simulink model "Prj2CDig"  (R2026a)
settings: Solver=ode45  StopTime=3600  RelTol=1e-6  EnableMultiTasking=on
values from neighbouring files (symbols this model uses):
  A = (Tz-Tp1)/(Tp2-Tp1)    (= 0.157044591698)    [Prj2CDig_m.m]
  B = 1 - A    (= 0.842955408302)    [Prj2CDig_m.m]
  K = Ka(1:2)    [Prj2CDig_m.m]
  Ki = -Ka(3)    [Prj2CDig_m.m]
  Kp = 0.8864/256.0    (= 0.0034625)    [Prj2CDig_m.m]
  L = acker(Aa',Ca',o)    [Prj2CDig_m.m]
  Nb = -Ki/p(1)    [Prj2CDig_m.m]
  PO = 60    [Prj2CDig_m.m]
  Ta = 27.4    [Prj2CDig_m.m]
  Tp1 = 323.16    [Prj2CDig_m.m]
  Tp2 = 37.636    [Prj2CDig_m.m]
  w0 = 0.09817477042468    (= 0.0981747704247)    [Prj2CDig_m.m]
  x1ei = 0    [Prj2CDig_m.m]
  x1i = 0    [Prj2CDig_m.m]
  x2ei = 0    [Prj2CDig_m.m]
  x2i = 0    [Prj2CDig_m.m]
  xii = 0    [Prj2CDig_m.m]
  xs1i = 0    [Prj2CDig_m.m]
  xs2i = 0    [Prj2CDig_m.m]
settings Model: Creator=Adolfo  LastModifiedBy=pedro
settings SolverCC: ZeroCrossControl=DisableAll
settings DataIOCC: MaxDataPoints=25000  SignalLoggingSaveFormat=ModelDataLogs
settings OptimizationCC: BooleanDataType=off  InitFltsAndDblsToZero=on
settings DebuggingCC: SaveWithParameterizedLinksMsg=none  UnderspecifiedInitializationDetection=Classic  SignalResolutionControl=TryResolveAllWithWarning  MultiTaskDSMMsg=warning  MultiTaskCondExecSysMsg=none
settings HardwareCC: ProdHWDeviceType=32-bit Generic  TargetUnknown=on
settings GRTTargetCC: TargetFcnLib=ansi_tfl_tmw.mat  CombineOutputUpdateFcns=off  GRTInterface=on

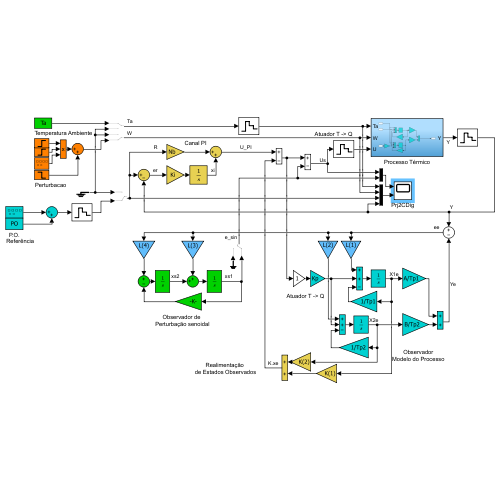
[thumbnail: Simulink's stored preview of the top-level diagram]
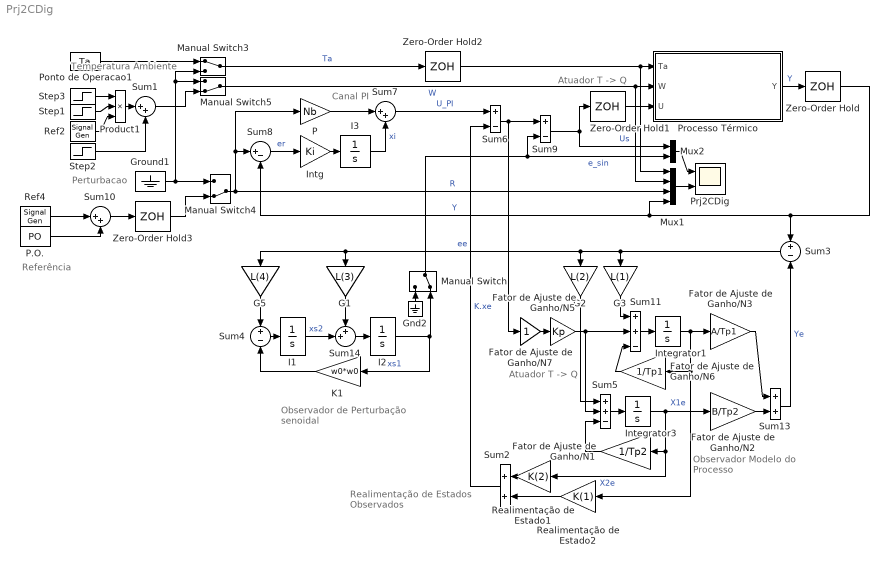
== system Prj2CDig ==
  note: Temperatura Ambiente
  note: Atuador T -> Q
  note: Referência
  note: Perturbacao
  note: Realimentação
      | de Estados Observados
  note: Observador de
      | Perturbação senoidal
  note: Observador
      | Modelo do Processo
  note: Canal PI
  note: Atuador T -> Q
  Fator de Ajuste de Ganho/N1 : Gain  Gain=1/Tp2  SaturateOnIntegerOverflow=on  OutDataTypeStr=Inherit: Same as input  ParamDataTypeStr=Inherit: Same as input
  Fator de Ajuste de Ganho/N2 : Gain  Gain=B/Tp2  SaturateOnIntegerOverflow=on  OutDataTypeStr=Inherit: Same as input  ParamDataTypeStr=Inherit: Same as input
  Fator de Ajuste de Ganho/N3 : Gain  Gain=A/Tp1  SaturateOnIntegerOverflow=on  OutDataTypeStr=Inherit: Same as input  ParamDataTypeStr=Inherit: Same as input
  Fator de Ajuste de Ganho/N5 : Gain  Gain=Kp  SaturateOnIntegerOverflow=on  OutDataTypeStr=Inherit: Same as input  ParamDataTypeStr=Inherit: Same as input
  Fator de Ajuste de Ganho/N6 : Gain  Gain=1/Tp1  SaturateOnIntegerOverflow=on  OutDataTypeStr=Inherit: Same as input  ParamDataTypeStr=Inherit: Same as input
  Fator de Ajuste de Ganho/N7 : Gain  SaturateOnIntegerOverflow=on  OutDataTypeStr=Inherit: Same as input  ParamDataTypeStr=Inherit: Same as input
  G1 : Gain  Gain=L(3)  SaturateOnIntegerOverflow=on  OutDataTypeStr=Inherit: Same as input  ParamDataTypeStr=Inherit: Same as input
  G2 : Gain  Gain=L(2)  SaturateOnIntegerOverflow=on  OutDataTypeStr=Inherit: Same as input  ParamDataTypeStr=Inherit: Same as input
  G3 : Gain  Gain=L(1)  SaturateOnIntegerOverflow=on  OutDataTypeStr=Inherit: Same as input  ParamDataTypeStr=Inherit: Same as input
  G5 : Gain  Gain=L(4)  SaturateOnIntegerOverflow=on  OutDataTypeStr=Inherit: Same as input  ParamDataTypeStr=Inherit: Same as input
  Gnd2 : Ground
  Ground1 : Ground
  I1 : Integrator  InitialCondition=xs2i
  I2 : Integrator  InitialCondition=xs1i
  I3 : Integrator  InitialCondition=xii
  Integrator1 : Integrator  InitialCondition=x1ei
  Integrator3 : Integrator  InitialCondition=x2ei
  Intg : Gain  Gain=Ki
  K1 : Gain  Gain=w0*w0  SaturateOnIntegerOverflow=on  OutDataTypeStr=Inherit: Same as input  ParamDataTypeStr=Inherit: Same as input
  Manual Switch : ManualSwitch  CurrentSetting=0
  Manual Switch3 : ManualSwitch
  Manual Switch4 : ManualSwitch  CurrentSetting=0
  Manual Switch5 : ManualSwitch  CurrentSetting=0
  Mux1 : Mux
  Mux2 : Mux  Inputs=2
  P : Gain  Gain=Nb
  P.O. : Constant  Value=PO
  Ponto de Operacao1 : Constant  Value=Ta
  Prj2CDig : Scope  NumInputPorts=2
      settings: TimeSpan=3600  ActiveDisplayYMinimum=-36403.221663907687  ActiveDisplayYMaximum=68827.440486001709  DataLoggingMaxPoints=30000
  Processo Térmico : Subsystem
  Product1 : Product  Inputs=3  RndMeth=Zero
  Realimentação de Estado1 : Gain  Gain=K(2)  SaturateOnIntegerOverflow=on  OutDataTypeStr=Inherit: Same as input  ParamDataTypeStr=Inherit: Same as input
  Realimentação de Estado2 : Gain  Gain=K(1)  SaturateOnIntegerOverflow=on  OutDataTypeStr=Inherit: Same as input  ParamDataTypeStr=Inherit: Same as input
  Ref2 : SignalGenerator  Frequency=w0  Units=rad/sec
  Ref4 : SignalGenerator  WaveForm=square  Amplitude=5  Frequency=.00125
  Step1 : Step  Time=3000  InitialValue=-20  FinalValue=0  SampleTime=0
  Step2 : Step  Time=1000  FinalValue=-20  SampleTime=0
  Step3 : Step  Time=1800  SampleTime=0
  Sum1 : Sum  Inputs=|++
  Sum10 : Sum  Inputs=|++
  Sum11 : Sum  Inputs=++-
  Sum13 : Sum  InputSameDT=on  SaturateOnIntegerOverflow=on  OutDataTypeStr=Inherit: Same as first input
  Sum14 : Sum  Inputs=++|  InputSameDT=on  SaturateOnIntegerOverflow=on  OutDataTypeStr=Inherit: Same as first input
  Sum2 : Sum
  Sum{3..4,6,9} (4 alike) : Sum  Inputs=+-  InputSameDT=on  SaturateOnIntegerOverflow=on  OutDataTypeStr=Inherit: Same as first input
  Sum5 : Sum  Inputs=++-
  Sum7 : Sum  Inputs=|++
  Sum8 : Sum  Inputs=|+-
  Zero-Order Hold{,1..3} (4 alike) : ZeroOrderHold  SampleTime=5
  wires:
  Sum9/1 -> Zero-Order Hold1/1, Mux2/1  "Us"
  P.O./1 -> Sum10/2
  Intg/1 -> I3/1
  Sum8/1 -> Intg/1  "er"
  P/1 -> Sum7/1
  I3/1 -> Sum7/2  "xi"
  Zero-Order Hold1/1 -> Processo Térmico/3(U)
  Manual Switch5/1 -> Mux1/2, Processo Térmico/2(W)  "W"
  Manual Switch3/1 -> Zero-Order Hold2/1  "Ta"
  Ground1/1 -> Manual Switch3/2, Manual Switch5/1, Manual Switch4/1
  Manual Switch4/1 -> Sum8/1, P/1, Mux1/3  "R"
  Sum1/1 -> Manual Switch5/2
  Ponto de Operacao1/1 -> Manual Switch3/1
  Sum10/1 -> Zero-Order Hold3/1
  Step2/1 -> Sum1/2
  Product1/1 -> Sum1/1
  Zero-Order Hold/1 -> Sum3/1, Sum8/2, Mux1/4  "Y"
  Fator de Ajuste de Ganho/N1/1 -> Sum5/3
  Integrator1/1 -> Fator de Ajuste de Ganho/N3/1, Fator de Ajuste de Ganho/N6/1, Realimentação de Estado2/1  "X1e"
  Manual Switch/1 -> Mux2/2, Sum9/2  "e_sin"
  Sum2/1 -> Sum6/2  "K.xe"
  Fator de Ajuste de Ganho/N6/1 -> Sum11/3
  Sum3/1 -> G5/1, G1/1, G2/1, G3/1  "ee"
  K1/1 -> Sum4/2
  Realimentação de Estado1/1 -> Sum2/1
  G5/1 -> Sum4/1
  I2/1 -> Manual Switch/2, K1/1  "xs1"
  Sum11/1 -> Integrator1/1
  Fator de Ajuste de Ganho/N2/1 -> Sum13/2
  Realimentação de Estado2/1 -> Sum2/2
  Sum5/1 -> Integrator3/1
  G3/1 -> Sum11/1
  Integrator3/1 -> Fator de Ajuste de Ganho/N2/1, Fator de Ajuste de Ganho/N1/1, Realimentação de Estado1/1  "X2e"
  Sum4/1 -> I1/1
  G2/1 -> Sum5/1
  Sum7/1 -> Sum6/1  "U_PI"
  Fator de Ajuste de Ganho/N5/1 -> Sum5/2, Sum11/2
  Sum14/1 -> I2/1
  I1/1 -> Sum14/2  "xs2"
  G1/1 -> Sum14/1
  Sum13/1 -> Sum3/2  "Ye"
  Fator de Ajuste de Ganho/N3/1 -> Sum13/1
  Sum6/1 -> Sum9/1, Fator de Ajuste de Ganho/N7/1
  Ref4/1 -> Sum10/1
  Gnd2/1 -> Manual Switch/1
  Mux1/1 -> Prj2CDig/2
  Fator de Ajuste de Ganho/N7/1 -> Fator de Ajuste de Ganho/N5/1
  Mux2/1 -> Prj2CDig/1
  Ref2/1 -> Product1/3
  Step1/1 -> Product1/2
  Step3/1 -> Product1/1
  Processo Térmico/1(Y) -> Zero-Order Hold/1  "Y"
  Zero-Order Hold2/1 -> Mux1/1, Processo Térmico/1(Ta)
  Zero-Order Hold3/1 -> Manual Switch4/2

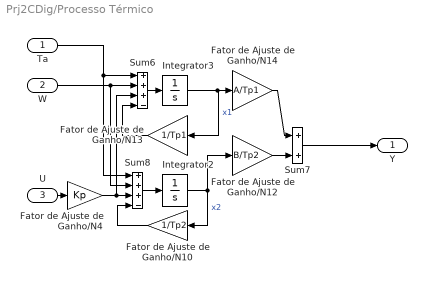
== system Prj2CDig/Processo Térmico ==
  Ta : Inport
  W : Inport  Port=2
  U : Inport  Port=3
  Fator de Ajuste de Ganho/N10 : Gain  Gain=1/Tp2  SaturateOnIntegerOverflow=on  OutDataTypeStr=Inherit: Same as input  ParamDataTypeStr=Inherit: Same as input
  Fator de Ajuste de Ganho/N12 : Gain  Gain=B/Tp2  SaturateOnIntegerOverflow=on  OutDataTypeStr=Inherit: Same as input  ParamDataTypeStr=Inherit: Same as input
  Fator de Ajuste de Ganho/N13 : Gain  Gain=1/Tp1  SaturateOnIntegerOverflow=on  OutDataTypeStr=Inherit: Same as input  ParamDataTypeStr=Inherit: Same as input
  Fator de Ajuste de Ganho/N14 : Gain  Gain=A/Tp1  SaturateOnIntegerOverflow=on  OutDataTypeStr=Inherit: Same as input  ParamDataTypeStr=Inherit: Same as input
  Fator de Ajuste de Ganho/N4 : Gain  Gain=Kp  SaturateOnIntegerOverflow=on  OutDataTypeStr=Inherit: Same as input  ParamDataTypeStr=Inherit: Same as input
  Integrator2 : Integrator  InitialCondition=x2i
  Integrator3 : Integrator  InitialCondition=x1i
  Sum6 : Sum  Inputs=+++-
  Sum7 : Sum  InputSameDT=on  SaturateOnIntegerOverflow=on  OutDataTypeStr=Inherit: Same as first input
  Sum8 : Sum  Inputs=+++-
  Y : Outport
  wires:
  Fator de Ajuste de Ganho/N12/1 -> Sum7/2
  Fator de Ajuste de Ganho/N13/1 -> Sum6/4
  Sum8/1 -> Integrator2/1
  Sum6/1 -> Integrator3/1
  Fator de Ajuste de Ganho/N10/1 -> Sum8/4
  U/1 -> Fator de Ajuste de Ganho/N4/1
  Fator de Ajuste de Ganho/N14/1 -> Sum7/1
  Integrator3/1 -> Fator de Ajuste de Ganho/N14/1, Fator de Ajuste de Ganho/N13/1  "x1"
  Integrator2/1 -> Fator de Ajuste de Ganho/N12/1, Fator de Ajuste de Ganho/N10/1  "x2"
  Ta/1 -> Sum8/1, Sum6/1
  Fator de Ajuste de Ganho/N4/1 -> Sum6/3, Sum8/3
  W/1 -> Sum8/2, Sum6/2
  Sum7/1 -> Y/1
